simulink model "chap05"  (R2021a)
settings: Solver=FixedStepDiscrete  StartTime=0.0  StopTime=inf  FixedStep=0.001  RelTol=1e-3
undefined symbols (not defined in the file): DiscIntNeverNeededParam, Header, Pose, X, Y, Z
libraries: robotlib x31
(part 6 of 9)

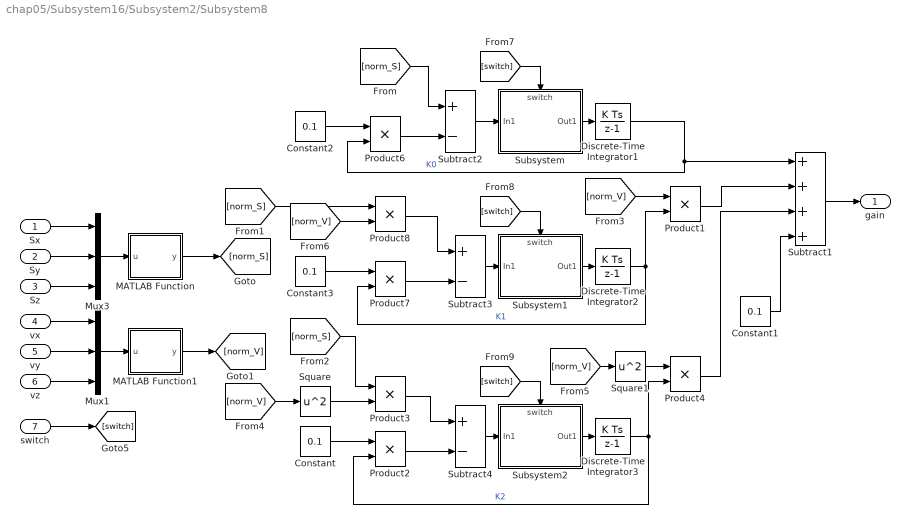
== system chap05/Subsystem16/Subsystem2/Subsystem8 ==
  Sx : Inport
  Sy : Inport  Port=2
  Sz : Inport  Port=3
  vx : Inport  Port=4
  vy : Inport  Port=5
  vz : Inport  Port=6
  switch : Inport  Port=7
  Constant{,1..3} (4 alike) : Constant  Value=0.1
  Discrete-Time Integrator1 : DiscreteIntegrator  gainval=1  InitialCondition=0.05  SampleTime=-1  ICPrevOutput=DiscIntNeverNeededParam  ICPrevScaledInput=DiscIntNeverNeededParam
  Discrete-Time Integrator2 : DiscreteIntegrator  gainval=1  InitialCondition=0.025  SampleTime=-1  ICPrevOutput=DiscIntNeverNeededParam  ICPrevScaledInput=DiscIntNeverNeededParam
  Discrete-Time Integrator3 : DiscreteIntegrator  gainval=1  InitialCondition=0.01  SampleTime=-1  ICPrevOutput=DiscIntNeverNeededParam  ICPrevScaledInput=DiscIntNeverNeededParam
  MATLAB Function : MATLAB Function  TreatAsAtomicUnit=on
  MATLAB Function1 : MATLAB Function  TreatAsAtomicUnit=on
  Mux1 : Mux  Inputs=3
  Mux3 : Mux  Inputs=3
  Product{1..4,6..8} (7 alike) : Product
  Square : Math  Operator=square  SaturateOnIntegerOverflow=on
  Square1 : Math  Operator=square  SaturateOnIntegerOverflow=on
  Subsystem : Subsystem
      settings: PortSchema="{\"entries\":[{\"content\":{\"sides\":[{\"content\":{\"connectorIds\":[\"In1\"]},\"type\":\"ConnectorPlacement.EquallySpacedRectSide\",\"uuid\":\"50b1559e-7173-4ba8-93e6-314f6d9df527\"},{\"content\":{\"connectorIds\":[\"Out1\"],\"side\":\"RIGHT\"},\"type\":\"ConnectorPlacement.EquallySpacedRectSide\",\"uuid\":\"be527bac-0bcc-4faf-a185-0382edae0189\"},{\"content\":{\"connectorIds\":[\"In2\"],\"side\":\"TOP\"},\"type\":\"ConnectorPlacement.EquallySpacedRectSide\",\"uuid\":\"4c8ef68d-7cf5-4d15-9758-89dbc1169805\"}]},\"type\":\"ConnectorPlacement.EquallySpacedConnector\",\"uuid\":\"3c2ee67b-c3c9-431a-8107-6d5cd22b236e\"}],\"packageUris\":[\"http://schema.mathworks.com/mf0/Connector/R2020b\"],\"version\":\"1.0\"}"
  Subsystem1 : Subsystem
      settings: PortSchema="{\"entries\":[{\"content\":{\"sides\":[{\"content\":{\"connectorIds\":[\"In1\"]},\"type\":\"ConnectorPlacement.EquallySpacedRectSide\",\"uuid\":\"50b1559e-7173-4ba8-93e6-314f6d9df527\"},{\"content\":{\"connectorIds\":[\"Out1\"],\"side\":\"RIGHT\"},\"type\":\"ConnectorPlacement.EquallySpacedRectSide\",\"uuid\":\"be527bac-0bcc-4faf-a185-0382edae0189\"},{\"content\":{\"connectorIds\":[\"In2\"],\"side\":\"TOP\"},\"type\":\"ConnectorPlacement.EquallySpacedRectSide\",\"uuid\":\"4c8ef68d-7cf5-4d15-9758-89dbc1169805\"}]},\"type\":\"ConnectorPlacement.EquallySpacedConnector\",\"uuid\":\"3c2ee67b-c3c9-431a-8107-6d5cd22b236e\"}],\"packageUris\":[\"http://schema.mathworks.com/mf0/Connector/R2020b\"],\"version\":\"1.0\"}"
  Subsystem2 : Subsystem
      settings: PortSchema="{\"entries\":[{\"content\":{\"sides\":[{\"content\":{\"connectorIds\":[\"In1\"]},\"type\":\"ConnectorPlacement.EquallySpacedRectSide\",\"uuid\":\"50b1559e-7173-4ba8-93e6-314f6d9df527\"},{\"content\":{\"connectorIds\":[\"Out1\"],\"side\":\"RIGHT\"},\"type\":\"ConnectorPlacement.EquallySpacedRectSide\",\"uuid\":\"be527bac-0bcc-4faf-a185-0382edae0189\"},{\"content\":{\"connectorIds\":[\"In2\"],\"side\":\"TOP\"},\"type\":\"ConnectorPlacement.EquallySpacedRectSide\",\"uuid\":\"4c8ef68d-7cf5-4d15-9758-89dbc1169805\"}]},\"type\":\"ConnectorPlacement.EquallySpacedConnector\",\"uuid\":\"3c2ee67b-c3c9-431a-8107-6d5cd22b236e\"}],\"packageUris\":[\"http://schema.mathworks.com/mf0/Connector/R2020b\"],\"version\":\"1.0\"}"
  Subtract1 : Sum  Inputs=++++
  Subtract2 : Sum  Inputs=+-
  Subtract3 : Sum  Inputs=+-
  Subtract4 : Sum  Inputs=+-
  " gain" : Outport
  wires:
  [switch] -> Subsystem2/2(switch)
  [switch] -> Subsystem1/2(switch)
  [switch] -> Subsystem/2(switch)
  switch/1 -> [switch]
  Subsystem1/1(Out1) -> Discrete-Time Integrator2/1
  Subsystem2/1(Out1) -> Discrete-Time Integrator3/1
  Subsystem/1(Out1) -> Discrete-Time Integrator1/1
  [norm_V] -> Product8/2
  Square1/1 -> Product4/1
  [norm_V] -> Square1/1
  [norm_V] -> Product1/1
  [norm_V] -> Square/1
  [norm_S] -> Product3/1
  [norm_S] -> Product8/1
  [norm_S] -> Subtract2/1
  MATLAB Function/1(y) -> [norm_S]
  vy/1 -> Mux1/2
  vz/1 -> Mux1/3
  vx/1 -> Mux1/1
  Sz/1 -> Mux3/3
  Sy/1 -> Mux3/2
  Sx/1 -> Mux3/1
  Constant3/1 -> Product7/1
  Constant2/1 -> Product6/1
  Constant1/1 -> Subtract1/4
  Product4/1 -> Subtract1/3
  MATLAB Function1/1(y) -> [norm_V]
  Constant/1 -> Product2/1
  Mux1/1 -> MATLAB Function1/1(u)
  Square/1 -> Product3/2
  Mux3/1 -> MATLAB Function/1(u)
  Discrete-Time Integrator3/1 -> Product2/2, Product4/2  "K2"
  Product2/1 -> Subtract4/2
  Product3/1 -> Subtract4/1
  Subtract4/1 -> Subsystem2/1(In1)
  Subtract3/1 -> Subsystem1/1(In1)
  Product8/1 -> Subtract3/1
  Product7/1 -> Subtract3/2
  Discrete-Time Integrator2/1 -> Product1/2, Product7/2  "K1"
  Product6/1 -> Subtract2/2
  Discrete-Time Integrator1/1 -> Subtract1/1, Product6/2  "K0"
  Subtract2/1 -> Subsystem/1(In1)
  Product1/1 -> Subtract1/2
  Subtract1/1 -> " gain"/1

== system chap05/Subsystem16/Subsystem2/Subsystem9 ==
  vy2 : Inport
  uty : Inport  Port=2
  gain : Inport  Port=3
  switch : Inport  Port=4
  Add1 : Sum  Inputs=--+
  Constant1 : Constant  Value=0.08
  Constant2 : Constant  Value=10
  Product : Product
  Product1 : Product
  Product2 : Product
  Subsystem : Subsystem
  Subtract : Sum  Inputs=+-
  Switch1 : Switch  Criteria=u2 > Threshold  Threshold=1
  Tanh : Trigonometry  Operator=tanh
  uy : Outport
  Sz : Outport  Port=2
  wires:
  Switch1/1 -> uy/1
  [switch] -> Switch1/2
  [A] -> Switch1/3
  switch/1 -> Subsystem/1(switch), [switch]
  Subtract/1 -> Product2/1, Product1/2, Sz/1
  Product1/1 -> Add1/1
  Constant2/1 -> Product2/2
  [A] -> Add1/3
  gain/1 -> Product/2
  Tanh/1 -> Product/1
  Product2/1 -> Tanh/1
  vy2/1 -> Subtract/1
  Product/1 -> Add1/2
  uty/1 -> Subsystem/2(zt3), [A]
  Add1/1 -> Switch1/1
  Subsystem/1(Out1) -> Subtract/2
  Constant1/1 -> Product1/1

== system chap05/Subsystem16/Subsystem3/Subsystem1 ==
  xy4 : Inport
  xy2 : Inport  Port=2
  xy3 : Inport  Port=3
  xy5 : Inport  Port=4
  vy4 : Inport  Port=5
  vy2 : Inport  Port=6
  vy3 : Inport  Port=7
  vy5 : Inport  Port=8
  Add : Sum
  Add{1,4,6,8} (4 alike) : Sum  Inputs=-+
  Add2 : Sum  Inputs=+-
  Add5 : Sum  Inputs=+++
  Add7 : Sum  Inputs=+-
  Add9 : Sum  Inputs=+++
  Constant : Constant  Value=0.75
  Constant1 : Constant  Value=0.85
  Constant2 : Constant  Value=0.8
  Constant3 : Constant  Value=0.8
  Constant4 : Constant  Value=0.5
  Constant5 : Constant  Value=1.2
  Constant6 : Constant  Value=0.5
  Constant7 : Constant  Value=1.2
  Gain : Gain  Gain=-1
  Product{1,3..9} (8 alike) : Product
  utx : Outport
  wires:
  Add9/1 -> Product1/2
  Product4/1 -> Add5/2
  Product5/1 -> Add5/3
  Constant3/1 -> Product4/1
  Add4/1 -> Product4/2
  xy4/1 -> Add1/2, Add4/2, Add2/1
  Constant4/1 -> Product5/2
  Product6/1 -> Add/1
  Constant/1 -> Product6/1
  Constant1/1 -> Product1/1
  Product1/1 -> Add/2
  Add2/1 -> Product5/1
  Add5/1 -> Product6/2
  xy3/1 -> Add4/1
  xy2/1 -> Add2/2
  xy5/1 -> Add1/1
  Constant5/1 -> Product3/1
  Add1/1 -> Product3/2
  Product3/1 -> Add5/1
  Product7/1 -> Add9/1
  Add6/1 -> Product7/2
  Constant7/1 -> Product7/1
  vy5/1 -> Add6/1
  vy2/1 -> Add7/2
  vy3/1 -> Add8/1
  Add7/1 -> Product9/1
  Constant6/1 -> Product9/2
  vy4/1 -> Add7/1, Add8/2, Add6/2
  Add8/1 -> Product8/2
  Constant2/1 -> Product8/1
  Product9/1 -> Add9/3
  Product8/1 -> Add9/2
  Gain/1 -> utx/1
  Add/1 -> Gain/1

== system chap05/Subsystem16/Subsystem3/Subsystem10 ==
  utx : Inport
  uty : Inport  Port=2
  utz : Inport  Port=3
  Add : Sum
  Constant3 : Constant
  Constant4 : Constant  Value=0
  Data Store Memory : DataStoreMemory  DataStoreName=utkz4  ReadBeforeWriteMsg=warning  WriteAfterWriteMsg=warning  WriteAfterReadMsg=warning  ShowAdditionalParam=off
  Data Store Memory1 : DataStoreMemory  DataStoreName=utky4  ReadBeforeWriteMsg=warning  WriteAfterWriteMsg=warning  WriteAfterReadMsg=warning  ShowAdditionalParam=off
  Data Store Memory2 : DataStoreMemory  DataStoreName=utkx4  ReadBeforeWriteMsg=warning  WriteAfterWriteMsg=warning  WriteAfterReadMsg=warning  ShowAdditionalParam=off
  Data Store Memory3 : DataStoreMemory  DataStoreName=uc4  ReadBeforeWriteMsg=warning  WriteAfterWriteMsg=warning  WriteAfterReadMsg=warning  ShowAdditionalParam=off
  Data Store Read : DataStoreRead  DataStoreName=uc4  IndexOptions=Index vector (dialog)  Indices=1  OutputSizes=1
  Data Store Read1 : DataStoreRead  DataStoreName=utkz4  IndexOptions=Index vector (dialog)  Indices=1  OutputSizes=1
  Data Store Read2 : DataStoreRead  DataStoreName=utky4  IndexOptions=Index vector (dialog)  Indices=1  OutputSizes=1
  Data Store Read3 : DataStoreRead  DataStoreName=utkx4  IndexOptions=Index vector (dialog)  Indices=1  OutputSizes=1
  Data Store Write : DataStoreWrite  DataStoreName=uc4  IndexOptions=Index vector (dialog)  Indices=1  OutputSizes=1
  Data Store Write3 : DataStoreWrite  DataStoreName=utkx4  IndexOptions=Index vector (dialog)  Indices=1  OutputSizes=1
  Data Store Write4 : DataStoreWrite  DataStoreName=utky4  IndexOptions=Index vector (dialog)  Indices=1  OutputSizes=1
  Data Store Write5 : DataStoreWrite  DataStoreName=utkz4  IndexOptions=Index vector (dialog)  Indices=1  OutputSizes=1
  Demux : Demux  Outputs=3
  Display : Display
  MATLAB Function : MATLAB Function  TreatAsAtomicUnit=on
  Mux1 : Mux  Inputs=3
  Mux2 : Mux  Inputs=3
  Switch : Switch  Threshold=0.1
  Switch2 : Switch  Threshold=0.1
  ux : Outport
  uy : Outport  Port=2
  uz : Outport  Port=3
  wires:
  Mux2/1 -> [utk], MATLAB Function/2(utk)
  Mux1/1 -> [ut], MATLAB Function/1(u)
  Switch/1 -> Demux/1
  Data Store Read3/1 -> Mux2/1
  Data Store Read1/1 -> Mux2/3
  Data Store Read2/1 -> Mux2/2
  Demux/3 -> Data Store Write5/1, uz/1
  Demux/1 -> Data Store Write3/1, ux/1
  Add/1 -> Data Store Write/1, Display/1
  Data Store Read/1 -> Add/2
  Switch2/1 -> Add/1  "e1"
  Constant3/1 -> Switch2/1
  Constant4/1 -> Switch2/3
  MATLAB Function/1(nrom) -> Switch2/2, Switch/2
  utx/1 -> Mux1/1
  uty/1 -> Mux1/2
  utz/1 -> Mux1/3
  Demux/2 -> Data Store Write4/1, uy/1
  [ut] -> Switch/1
  [utk] -> Switch/3

== system chap05/Subsystem16/Subsystem3/Subsystem11 ==
  vz4 : Inport
  utz : Inport  Port=2
  gain : Inport  Port=3
  switch : Inport  Port=4
  Add1 : Sum  Inputs=--+
  Constant1 : Constant  Value=0.08
  Constant2 : Constant  Value=10
  Product : Product
  Product1 : Product
  Product2 : Product
  Subsystem : Subsystem
  Subtract : Sum  Inputs=+-
  Switch1 : Switch  Criteria=u2 > Threshold  Threshold=1
  Tanh : Trigonometry  Operator=tanh
  uz : Outport
  Sz : Outport  Port=2
  wires:
  Add1/1 -> Switch1/1
  utz/1 -> [A], Subsystem/2(zt3)
  Product/1 -> Add1/2
  vz4/1 -> Subtract/1
  Product2/1 -> Tanh/1
  Tanh/1 -> Product/1
  gain/1 -> Product/2
  [A] -> Add1/3
  Constant2/1 -> Product2/2
  Product1/1 -> Add1/1
  Constant1/1 -> Product1/1
  Subtract/1 -> Sz/1, Product1/2, Product2/1
  Subsystem/1(Out1) -> Subtract/2
  switch/1 -> [switch], Subsystem/1(switch)
  [A] -> Switch1/3
  [switch] -> Switch1/2
  Switch1/1 -> uz/1

== system chap05/Subsystem16/Subsystem3/Subsystem2 ==
  xz4 : Inport
  xx2 : Inport  Port=2
  xz3 : Inport  Port=3
  xz5 : Inport  Port=4
  vz4 : Inport  Port=5
  vz2 : Inport  Port=6
  vz3 : Inport  Port=7
  vz5 : Inport  Port=8
  Add : Sum
  Add{1,4,6,8} (4 alike) : Sum  Inputs=-+
  Add2 : Sum  Inputs=+-
  Add5 : Sum  Inputs=+++
  Add7 : Sum  Inputs=+-
  Add9 : Sum  Inputs=+++
  Constant : Constant  Value=0.75
  Constant1 : Constant  Value=0.85
  Constant2 : Constant  Value=0.8
  Constant3 : Constant  Value=0.8
  Constant4 : Constant  Value=0.5
  Constant5 : Constant  Value=1.2
  Constant6 : Constant  Value=0.5
  Constant7 : Constant  Value=1.2
  Gain : Gain  Gain=-1
  Product{1,3..9} (8 alike) : Product
  utx : Outport
  wires:
  Product8/1 -> Add9/2
  Product9/1 -> Add9/3
  Constant2/1 -> Product8/1
  Add8/1 -> Product8/2
  vz4/1 -> Add6/2, Add8/2, Add7/1
  Constant6/1 -> Product9/2
  Add7/1 -> Product9/1
  vz3/1 -> Add8/1
  vz2/1 -> Add7/2
  vz5/1 -> Add6/1
  Constant7/1 -> Product7/1
  Add6/1 -> Product7/2
  Product7/1 -> Add9/1
  Product3/1 -> Add5/1
  Add1/1 -> Product3/2
  Constant5/1 -> Product3/1
  xz5/1 -> Add1/1
  xx2/1 -> Add2/2
  xz3/1 -> Add4/1
  Add5/1 -> Product6/2
  Add2/1 -> Product5/1
  Product1/1 -> Add/2
  Constant1/1 -> Product1/1
  Constant/1 -> Product6/1
  Product6/1 -> Add/1
  Constant4/1 -> Product5/2
  xz4/1 -> Add2/1, Add4/2, Add1/2
  Add4/1 -> Product4/2
  Constant3/1 -> Product4/1
  Product5/1 -> Add5/3
  Product4/1 -> Add5/2
  Add9/1 -> Product1/2
  Gain/1 -> utx/1
  Add/1 -> Gain/1

== system chap05/Subsystem16/Subsystem3/Subsystem3 ==
  utx : Inport
  vx : Inport  Port=2
  vy : Inport  Port=3
  vz : Inport  Port=4
  uty : Inport  Port=5
  ux : Inport  Port=6
  uy : Inport  Port=7
  uz : Inport  Port=8
  utz : Inport  Port=9
  switch : Inport  Port=10
  Add3 : Sum  Inputs=-+
  Add4 : Sum  Inputs=-+
  Add5 : Sum  Inputs=-+
  Demux : Demux  Outputs=3
  Demux1 : Demux  Outputs=3
  Discrete-Time Integrator1 : DiscreteIntegrator  SampleTime=-1  ICPrevOutput=DiscIntNeverNeededParam  ICPrevScaledInput=DiscIntNeverNeededParam
  Discrete-Time Integrator2 : DiscreteIntegrator  SampleTime=-1  ICPrevOutput=DiscIntNeverNeededParam  ICPrevScaledInput=DiscIntNeverNeededParam
  Discrete-Time Integrator8 : DiscreteIntegrator  SampleTime=-1  ICPrevOutput=DiscIntNeverNeededParam  ICPrevScaledInput=DiscIntNeverNeededParam
  MATLAB Function : MATLAB Function  TreatAsAtomicUnit=on
  MATLAB Function1 : MATLAB Function  TreatAsAtomicUnit=on
  MATLAB Function2 : MATLAB Function  TreatAsAtomicUnit=on
  Mux : Mux  Inputs=3
  Mux1 : Mux  Inputs=3
  Subsystem : Subsystem
  Subsystem1 : Subsystem
  Subsystem2 : Subsystem
      settings: PortSchema="{\"entries\":[{\"content\":{\"sides\":[{\"content\":{\"connectorIds\":[\"In1\"]},\"type\":\"ConnectorPlacement.EquallySpacedRectSide\",\"uuid\":\"fc08b57d-5108-4bb3-894e-d1527c9ee9b9\"},{\"content\":{\"connectorIds\":[\"Out1\",\"Out2\",\"Out3\",\"Out4\"],\"side\":\"RIGHT\"},\"type\":\"ConnectorPlacement.EquallySpacedRectSide\",\"uuid\":\"5f28f464-9d6d-4ee7-848e-113b4b51ead6\"},{\"content\":{\"connectorIds\":[],\"side\":\"TOP\"},\"type\":\"ConnectorPlacement.EquallySpacedRectSide\",\"uuid\":\"5cca314e-822b-43eb-ac4d-78622e8ed582\"},{\"content\":{\"connectorIds\":[\"In2\"],\"side\":\"BOTTOM\"},\"type\":\"ConnectorPlacement.EquallySpacedRectSide\",\"uuid\":\"aa07b2d0-4f6e-4d8e-96de-14c35ee3da88\"}]},\"type\":\"ConnectorPlacement.EquallySpacedConnector\",\"uuid\":\"246d6f2c-2f9e-403c-b810-eff9b0fc0735\"}],\"packageUris\":[\"http://schema.mathworks.com/mf0/Connector/R2020b\"],\"version\":\"1.0\"}"
  Subsystem3 : Subsystem
  Subtract1 : Sum  Inputs=++++
  Subtract2 : Sum  Inputs=+-
  Subtract3 : Sum  Inputs=+-
  Subtract4 : Sum  Inputs=+-
  Switch1 : Switch  Criteria=u2 > Threshold  Threshold=1
  Switch2 : Switch  Criteria=u2 > Threshold  Threshold=1
  Switch3 : Switch  Criteria=u2 > Threshold  Threshold=1
  udtx : Outport
  udty : Outport  Port=2
  udtz : Outport  Port=3
  wires:
  Subsystem3/1(Out1) -> Subtract1/2
  Subsystem2/2(k2) -> Subsystem3/2(k2)
  Subsystem1/1(Out1) -> Subtract1/1
  Subsystem2/1(k1) -> Subsystem1/2(k1)
  Subtract4/1 -> MATLAB Function2/1(u)
  Subtract3/1 -> MATLAB Function1/1(u)
  Subtract2/1 -> MATLAB Function/1(u)
  Demux/3 -> Discrete-Time Integrator8/1
  Demux/1 -> Discrete-Time Integrator2/1
  Demux/2 -> Discrete-Time Integrator1/1
  Discrete-Time Integrator2/1 -> Subtract2/1
  Discrete-Time Integrator1/1 -> Subtract3/1
  Discrete-Time Integrator8/1 -> Subtract4/1
  Mux1/1 -> Subtract1/4
  ux/1 -> Mux1/1
  uy/1 -> Mux1/2
  uz/1 -> Mux1/3
  vx/1 -> Subtract2/2
  Subsystem2/4(k4) -> Subsystem/3(k4)
  Subsystem/1(z2) -> Subtract1/3, Demux1/1  "od4"
  Subsystem2/3(k3) -> Subsystem/2(k3)
  Subtract1/1 -> Demux/1
  Mux/1 -> Subsystem1/1(e1), Subsystem3/1(e1), Subsystem2/1(e1), Subsystem/1(e1)
  utx/1 -> Switch1/3, Add3/2
  uty/1 -> Switch2/3, Add5/2
  utz/1 -> Switch3/3, Add4/2
  vy/1 -> Subtract3/2
  vz/1 -> Subtract4/2
  MATLAB Function/1(y) -> Mux/1
  MATLAB Function1/1(y) -> Mux/2
  MATLAB Function2/1(y) -> Mux/3
  switch/1 -> [switch], Switch3/2, Switch2/2, Switch1/2
  [switch] -> Subsystem2/2(switch)
  Add3/1 -> Switch1/1
  Add5/1 -> Switch2/1
  Add4/1 -> Switch3/1
  Switch1/1 -> udtx/1
  Switch2/1 -> udty/1
  Switch3/1 -> udtz/1
  Demux1/1 -> Add3/1
  Demux1/2 -> Add5/1
  Demux1/3 -> Add4/1

== system chap05/Subsystem16/Subsystem3/Subsystem4 ==
  vx4 : Inport
  utx : Inport  Port=2
  gain : Inport  Port=3
  switch : Inport  Port=4
  Add1 : Sum  Inputs=--+
  Constant1 : Constant  Value=0.08
  Constant2 : Constant  Value=10
  Product : Product
  Product1 : Product
  Product2 : Product
  Subsystem : Subsystem
  Subtract : Sum  Inputs=+-
  Switch1 : Switch  Criteria=u2 > Threshold  Threshold=1
  Tanh : Trigonometry  Operator=tanh
  ux : Outport
  Sx : Outport  Port=2
  wires:
  Add1/1 -> Switch1/1
  utx/1 -> [A], Subsystem/2(zt3)
  Product/1 -> Add1/2
  vx4/1 -> Subtract/1
  Product2/1 -> Tanh/1
  Tanh/1 -> Product/1
  gain/1 -> Product/2
  [A] -> Add1/3
  Constant2/1 -> Product2/2
  Product1/1 -> Add1/1
  Constant1/1 -> Product1/1
  Subtract/1 -> Sx/1, Product1/2, Product2/1
  switch/1 -> [switch], Subsystem/1(switch)
  [A] -> Switch1/3
  [switch] -> Switch1/2
  Switch1/1 -> ux/1
  Subsystem/1(Out1) -> Subtract/2

== system chap05/Subsystem16/Subsystem3/Subsystem6 ==
  xx4 : Inport
  xx2 : Inport  Port=2
  xx3 : Inport  Port=3
  xx5 : Inport  Port=4
  vx4 : Inport  Port=5
  vx2 : Inport  Port=6
  vx3 : Inport  Port=7
  vx5 : Inport  Port=8
  Add : Sum
  Add{1,4,6,8} (4 alike) : Sum  Inputs=-+
  Add2 : Sum  Inputs=+-
  Add5 : Sum  Inputs=+++
  Add7 : Sum  Inputs=+-
  Add9 : Sum  Inputs=+++
  Constant : Constant  Value=0.75
  Constant1 : Constant  Value=0.85
  Constant2 : Constant  Value=0.8
  Constant3 : Constant  Value=0.8
  Constant4 : Constant  Value=0.5
  Constant5 : Constant  Value=1.2
  Constant6 : Constant  Value=0.5
  Constant7 : Constant  Value=1.2
  Gain : Gain  Gain=-1
  Product{1,3..9} (8 alike) : Product
  utx : Outport
  wires:
  Product8/1 -> Add9/2
  Product9/1 -> Add9/3
  Constant2/1 -> Product8/1
  Add8/1 -> Product8/2
  vx4/1 -> Add6/2, Add8/2, Add7/1
  Constant6/1 -> Product9/2
  Add7/1 -> Product9/1
  vx3/1 -> Add8/1
  vx2/1 -> Add7/2
  vx5/1 -> Add6/1
  Constant7/1 -> Product7/1
  Add6/1 -> Product7/2
  Product7/1 -> Add9/1
  Product3/1 -> Add5/1
  Add1/1 -> Product3/2
  Constant5/1 -> Product3/1
  xx5/1 -> Add1/1
  xx2/1 -> Add2/2
  xx3/1 -> Add4/1
  Add5/1 -> Product6/2
  Add2/1 -> Product5/1
  Product1/1 -> Add/2
  Constant1/1 -> Product1/1
  Constant/1 -> Product6/1
  Product6/1 -> Add/1
  Constant4/1 -> Product5/2
  xx4/1 -> Add2/1, Add4/2, Add1/2
  Add4/1 -> Product4/2
  Constant3/1 -> Product4/1
  Product5/1 -> Add5/3
  Product4/1 -> Add5/2
  Add9/1 -> Product1/2
  Gain/1 -> utx/1
  Add/1 -> Gain/1

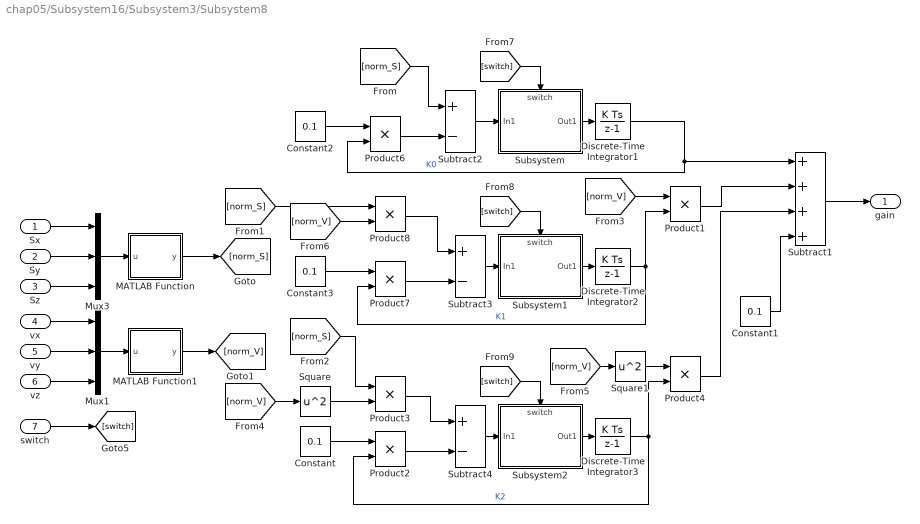
== system chap05/Subsystem16/Subsystem3/Subsystem8 ==
  Sx : Inport
  Sy : Inport  Port=2
  Sz : Inport  Port=3
  vx : Inport  Port=4
  vy : Inport  Port=5
  vz : Inport  Port=6
  switch : Inport  Port=7
  Constant{,1..3} (4 alike) : Constant  Value=0.1
  Discrete-Time Integrator1 : DiscreteIntegrator  gainval=1  InitialCondition=0.05  SampleTime=-1  ICPrevOutput=DiscIntNeverNeededParam  ICPrevScaledInput=DiscIntNeverNeededParam
  Discrete-Time Integrator2 : DiscreteIntegrator  gainval=1  InitialCondition=0.025  SampleTime=-1  ICPrevOutput=DiscIntNeverNeededParam  ICPrevScaledInput=DiscIntNeverNeededParam
  Discrete-Time Integrator3 : DiscreteIntegrator  gainval=1  InitialCondition=0.01  SampleTime=-1  ICPrevOutput=DiscIntNeverNeededParam  ICPrevScaledInput=DiscIntNeverNeededParam
  MATLAB Function : MATLAB Function  TreatAsAtomicUnit=on
  MATLAB Function1 : MATLAB Function  TreatAsAtomicUnit=on
  Mux1 : Mux  Inputs=3
  Mux3 : Mux  Inputs=3
  Product{1..4,6..8} (7 alike) : Product
  Square : Math  Operator=square  SaturateOnIntegerOverflow=on
  Square1 : Math  Operator=square  SaturateOnIntegerOverflow=on
  Subsystem : Subsystem
      settings: PortSchema="{\"entries\":[{\"content\":{\"sides\":[{\"content\":{\"connectorIds\":[\"In1\"]},\"type\":\"ConnectorPlacement.EquallySpacedRectSide\",\"uuid\":\"50b1559e-7173-4ba8-93e6-314f6d9df527\"},{\"content\":{\"connectorIds\":[\"Out1\"],\"side\":\"RIGHT\"},\"type\":\"ConnectorPlacement.EquallySpacedRectSide\",\"uuid\":\"be527bac-0bcc-4faf-a185-0382edae0189\"},{\"content\":{\"connectorIds\":[\"In2\"],\"side\":\"TOP\"},\"type\":\"ConnectorPlacement.EquallySpacedRectSide\",\"uuid\":\"4c8ef68d-7cf5-4d15-9758-89dbc1169805\"}]},\"type\":\"ConnectorPlacement.EquallySpacedConnector\",\"uuid\":\"3c2ee67b-c3c9-431a-8107-6d5cd22b236e\"}],\"packageUris\":[\"http://schema.mathworks.com/mf0/Connector/R2020b\"],\"version\":\"1.0\"}"
  Subsystem1 : Subsystem
      settings: PortSchema="{\"entries\":[{\"content\":{\"sides\":[{\"content\":{\"connectorIds\":[\"In1\"]},\"type\":\"ConnectorPlacement.EquallySpacedRectSide\",\"uuid\":\"50b1559e-7173-4ba8-93e6-314f6d9df527\"},{\"content\":{\"connectorIds\":[\"Out1\"],\"side\":\"RIGHT\"},\"type\":\"ConnectorPlacement.EquallySpacedRectSide\",\"uuid\":\"be527bac-0bcc-4faf-a185-0382edae0189\"},{\"content\":{\"connectorIds\":[\"In2\"],\"side\":\"TOP\"},\"type\":\"ConnectorPlacement.EquallySpacedRectSide\",\"uuid\":\"4c8ef68d-7cf5-4d15-9758-89dbc1169805\"}]},\"type\":\"ConnectorPlacement.EquallySpacedConnector\",\"uuid\":\"3c2ee67b-c3c9-431a-8107-6d5cd22b236e\"}],\"packageUris\":[\"http://schema.mathworks.com/mf0/Connector/R2020b\"],\"version\":\"1.0\"}"
  Subsystem2 : Subsystem
      settings: PortSchema="{\"entries\":[{\"content\":{\"sides\":[{\"content\":{\"connectorIds\":[\"In1\"]},\"type\":\"ConnectorPlacement.EquallySpacedRectSide\",\"uuid\":\"50b1559e-7173-4ba8-93e6-314f6d9df527\"},{\"content\":{\"connectorIds\":[\"Out1\"],\"side\":\"RIGHT\"},\"type\":\"ConnectorPlacement.EquallySpacedRectSide\",\"uuid\":\"be527bac-0bcc-4faf-a185-0382edae0189\"},{\"content\":{\"connectorIds\":[\"In2\"],\"side\":\"TOP\"},\"type\":\"ConnectorPlacement.EquallySpacedRectSide\",\"uuid\":\"4c8ef68d-7cf5-4d15-9758-89dbc1169805\"}]},\"type\":\"ConnectorPlacement.EquallySpacedConnector\",\"uuid\":\"3c2ee67b-c3c9-431a-8107-6d5cd22b236e\"}],\"packageUris\":[\"http://schema.mathworks.com/mf0/Connector/R2020b\"],\"version\":\"1.0\"}"
  Subtract1 : Sum  Inputs=++++
  Subtract2 : Sum  Inputs=+-
  Subtract3 : Sum  Inputs=+-
  Subtract4 : Sum  Inputs=+-
  " gain" : Outport
  wires:
  [switch] -> Subsystem2/2(switch)
  [switch] -> Subsystem1/2(switch)
  [switch] -> Subsystem/2(switch)
  switch/1 -> [switch]
  Subsystem1/1(Out1) -> Discrete-Time Integrator2/1
  Subsystem2/1(Out1) -> Discrete-Time Integrator3/1
  Subsystem/1(Out1) -> Discrete-Time Integrator1/1
  [norm_V] -> Product8/2
  Square1/1 -> Product4/1
  [norm_V] -> Square1/1
  [norm_V] -> Product1/1
  [norm_V] -> Square/1
  [norm_S] -> Product3/1
  [norm_S] -> Product8/1
  [norm_S] -> Subtract2/1
  MATLAB Function/1(y) -> [norm_S]
  vy/1 -> Mux1/2
  vz/1 -> Mux1/3
  vx/1 -> Mux1/1
  Sz/1 -> Mux3/3
  Sy/1 -> Mux3/2
  Sx/1 -> Mux3/1
  Constant3/1 -> Product7/1
  Constant2/1 -> Product6/1
  Constant1/1 -> Subtract1/4
  Product4/1 -> Subtract1/3
  MATLAB Function1/1(y) -> [norm_V]
  Constant/1 -> Product2/1
  Mux1/1 -> MATLAB Function1/1(u)
  Square/1 -> Product3/2
  Mux3/1 -> MATLAB Function/1(u)
  Discrete-Time Integrator3/1 -> Product2/2, Product4/2  "K2"
  Product2/1 -> Subtract4/2
  Product3/1 -> Subtract4/1
  Subtract4/1 -> Subsystem2/1(In1)
  Subtract3/1 -> Subsystem1/1(In1)
  Product8/1 -> Subtract3/1
  Product7/1 -> Subtract3/2
  Discrete-Time Integrator2/1 -> Product1/2, Product7/2  "K1"
  Product6/1 -> Subtract2/2
  Discrete-Time Integrator1/1 -> Subtract1/1, Product6/2  "K0"
  Subtract2/1 -> Subsystem/1(In1)
  Product1/1 -> Subtract1/2
  Subtract1/1 -> " gain"/1

== system chap05/Subsystem16/Subsystem3/Subsystem9 ==
  vy4 : Inport
  uty : Inport  Port=2
  gain : Inport  Port=3
  switch : Inport  Port=4
  Add1 : Sum  Inputs=--+
  Constant1 : Constant  Value=0.08
  Constant2 : Constant  Value=10
  Product : Product
  Product1 : Product
  Product2 : Product
  Subsystem : Subsystem
  Subtract : Sum  Inputs=+-
  Switch1 : Switch  Criteria=u2 > Threshold  Threshold=1
  Tanh : Trigonometry  Operator=tanh
  uy : Outport
  Sz : Outport  Port=2
  wires:
  Switch1/1 -> uy/1
  [switch] -> Switch1/2
  [A] -> Switch1/3
  switch/1 -> Subsystem/1(switch), [switch]
  Subtract/1 -> Product2/1, Product1/2, Sz/1
  Constant1/1 -> Product1/1
  Product1/1 -> Add1/1
  Constant2/1 -> Product2/2
  [A] -> Add1/3
  gain/1 -> Product/2
  Tanh/1 -> Product/1
  Product2/1 -> Tanh/1
  vy4/1 -> Subtract/1
  Product/1 -> Add1/2
  uty/1 -> Subsystem/2(zt3), [A]
  Add1/1 -> Switch1/1
  Subsystem/1(Out1) -> Subtract/2

== system chap05/Subsystem16/Subsystem5/Subsystem1 ==
  xy3 : Inport
  xy1 : Inport  Port=2
  xy4 : Inport  Port=3
  xy5 : Inport  Port=4
  vy3 : Inport  Port=5
  vy1 : Inport  Port=6
  vy4 : Inport  Port=7
  vy5 : Inport  Port=8
  Add : Sum
  Add{1,4,6,8} (4 alike) : Sum  Inputs=-+
  Add2 : Sum  Inputs=+-
  Add5 : Sum  Inputs=+++
  Add7 : Sum  Inputs=+-
  Add9 : Sum  Inputs=+++
  Constant : Constant  Value=0.75
  Constant1 : Constant  Value=0.85
  Constant2 : Constant  Value=0.8
  Constant3 : Constant  Value=0.8
  Constant4 : Constant  Value=0.5
  Constant5 : Constant  Value=1.5
  Constant6 : Constant  Value=0.5
  Constant7 : Constant  Value=1.5
  Gain : Gain  Gain=-1
  Product{1,3..9} (8 alike) : Product
  p3y : Outport
  wires:
  Add9/1 -> Product1/2
  Product4/1 -> Add5/2
  Product5/1 -> Add5/3
  Constant3/1 -> Product4/1
  Add4/1 -> Product4/2
  xy3/1 -> Add1/2, Add4/2, Add2/1
  Constant4/1 -> Product5/2
  Product6/1 -> Add/1
  Constant/1 -> Product6/1
  Constant1/1 -> Product1/1
  Product1/1 -> Add/2
  Add2/1 -> Product5/1
  Add5/1 -> Product6/2
  xy4/1 -> Add4/1
  xy1/1 -> Add2/2
  xy5/1 -> Add1/1
  Constant5/1 -> Product3/1
  Add1/1 -> Product3/2
  Product3/1 -> Add5/1
  Product7/1 -> Add9/1
  Add6/1 -> Product7/2
  Constant7/1 -> Product7/1
  vy5/1 -> Add6/1
  vy1/1 -> Add7/2
  vy4/1 -> Add8/1
  Add7/1 -> Product9/1
  Constant6/1 -> Product9/2
  vy3/1 -> Add7/1, Add8/2, Add6/2
  Add8/1 -> Product8/2
  ? -> Product8/1
  Product9/1 -> Add9/3
  Product8/1 -> Add9/2
  Gain/1 -> p3y/1
  Add/1 -> Gain/1

== system chap05/Subsystem16/Subsystem5/Subsystem10 ==
  utx : Inport
  uty : Inport  Port=2
  utz : Inport  Port=3
  Add : Sum
  Constant3 : Constant
  Constant4 : Constant  Value=0
  Data Store Memory : DataStoreMemory  DataStoreName=utkz3  ReadBeforeWriteMsg=warning  WriteAfterWriteMsg=warning  WriteAfterReadMsg=warning  ShowAdditionalParam=off
  Data Store Memory1 : DataStoreMemory  DataStoreName=utky3  ReadBeforeWriteMsg=warning  WriteAfterWriteMsg=warning  WriteAfterReadMsg=warning  ShowAdditionalParam=off
  Data Store Memory2 : DataStoreMemory  DataStoreName=utkx3  ReadBeforeWriteMsg=warning  WriteAfterWriteMsg=warning  WriteAfterReadMsg=warning  ShowAdditionalParam=off
  Data Store Memory3 : DataStoreMemory  DataStoreName=uc3  ReadBeforeWriteMsg=warning  WriteAfterWriteMsg=warning  WriteAfterReadMsg=warning  ShowAdditionalParam=off
  Data Store Read : DataStoreRead  DataStoreName=uc3  IndexOptions=Index vector (dialog)  Indices=1  OutputSizes=1
  Data Store Read4 : DataStoreRead  DataStoreName=utky3  IndexOptions=Index vector (dialog)  Indices=1  OutputSizes=1
  Data Store Read5 : DataStoreRead  DataStoreName=utkz3  IndexOptions=Index vector (dialog)  Indices=1  OutputSizes=1
  Data Store Read6 : DataStoreRead  DataStoreName=utkx3  IndexOptions=Index vector (dialog)  Indices=1  OutputSizes=1
  Data Store Write : DataStoreWrite  DataStoreName=uc3  IndexOptions=Index vector (dialog)  Indices=1  OutputSizes=1
  Data Store Write1 : DataStoreWrite  DataStoreName=utkx3  IndexOptions=Index vector (dialog)  Indices=1  OutputSizes=1
  Data Store Write2 : DataStoreWrite  DataStoreName=utky3  IndexOptions=Index vector (dialog)  Indices=1  OutputSizes=1
  Data Store Write3 : DataStoreWrite  DataStoreName=utkz3  IndexOptions=Index vector (dialog)  Indices=1  OutputSizes=1
  Demux : Demux  Outputs=3
  Display : Display
  MATLAB Function : MATLAB Function  TreatAsAtomicUnit=on
  Mux1 : Mux  Inputs=3
  Mux2 : Mux  Inputs=3
  Switch : Switch  Threshold=0.1
  Switch2 : Switch  Threshold=0.1
  ux : Outport
  uy : Outport  Port=2
  uz : Outport  Port=3
  wires:
  Mux2/1 -> [utk], MATLAB Function/2(utk)
  Mux1/1 -> [ut], MATLAB Function/1(u)
  Switch/1 -> Demux/1
  Data Store Read6/1 -> Mux2/1
  Data Store Read5/1 -> Mux2/3
  Data Store Read4/1 -> Mux2/2
  Demux/3 -> Data Store Write3/1, uz/1
  Demux/1 -> Data Store Write1/1, ux/1
  Add/1 -> Data Store Write/1, Display/1
  Data Store Read/1 -> Add/2
  Switch2/1 -> Add/1  "e1"
  Constant3/1 -> Switch2/1
  Constant4/1 -> Switch2/3
  MATLAB Function/1(nrom) -> Switch2/2, Switch/2
  utx/1 -> Mux1/1
  uty/1 -> Mux1/2
  utz/1 -> Mux1/3
  Demux/2 -> Data Store Write2/1, uy/1
  [ut] -> Switch/1
  [utk] -> Switch/3

== system chap05/Subsystem16/Subsystem5/Subsystem11 ==
  vz3 : Inport
  utz : Inport  Port=2
  gain : Inport  Port=3
  switch : Inport  Port=4
  Add1 : Sum  Inputs=--+
  Constant1 : Constant  Value=0.08
  Constant2 : Constant  Value=10
  Product : Product
  Product1 : Product
  Product2 : Product
  Subsystem : Subsystem
  Subtract : Sum  Inputs=+-
  Switch1 : Switch  Criteria=u2 > Threshold  Threshold=1
  Tanh : Trigonometry  Operator=tanh
  uz : Outport
  Sz : Outport  Port=2
  wires:
  Add1/1 -> Switch1/1
  utz/1 -> [A], Subsystem/2(zt3)
  Product/1 -> Add1/2
  vz3/1 -> Subtract/1
  Product2/1 -> Tanh/1
  Tanh/1 -> Product/1
  gain/1 -> Product/2
  [A] -> Add1/3
  Constant2/1 -> Product2/2
  Product1/1 -> Add1/1
  Constant1/1 -> Product1/1
  Subtract/1 -> Sz/1, Product1/2, Product2/1
  Subsystem/1(Out1) -> Subtract/2
  switch/1 -> [switch], Subsystem/1(switch)
  [A] -> Switch1/3
  [switch] -> Switch1/2
  Switch1/1 -> uz/1

== system chap05/Subsystem16/Subsystem5/Subsystem2 ==
  xz3 : Inport
  xz1 : Inport  Port=2
  xz4 : Inport  Port=3
  xz5 : Inport  Port=4
  vz3 : Inport  Port=5
  vz1 : Inport  Port=6
  vz4 : Inport  Port=7
  vz5 : Inport  Port=8
  Add : Sum
  Add{1,4,6,8} (4 alike) : Sum  Inputs=-+
  Add2 : Sum  Inputs=+-
  Add5 : Sum  Inputs=+++
  Add7 : Sum  Inputs=+-
  Add9 : Sum  Inputs=+++
  Constant : Constant  Value=0.75
  Constant1 : Constant  Value=0.85
  Constant2 : Constant  Value=0.8
  Constant3 : Constant  Value=0.8
  Constant4 : Constant  Value=0.5
  Constant5 : Constant  Value=1.5
  Constant6 : Constant  Value=0.5
  Constant7 : Constant  Value=1.5
  Gain : Gain  Gain=-1
  Product{1,3..9} (8 alike) : Product
  p3z : Outport
  wires:
  Product8/1 -> Add9/2
  Product9/1 -> Add9/3
  Constant2/1 -> Product8/1
  Add8/1 -> Product8/2
  vz3/1 -> Add6/2, Add8/2, Add7/1
  Constant6/1 -> Product9/2
  Add7/1 -> Product9/1
  vz4/1 -> Add8/1
  vz1/1 -> Add7/2
  vz5/1 -> Add6/1
  Constant7/1 -> Product7/1
  Add6/1 -> Product7/2
  Product7/1 -> Add9/1
  Product3/1 -> Add5/1
  Add1/1 -> Product3/2
  Constant5/1 -> Product3/1
  xz5/1 -> Add1/1
  xz1/1 -> Add2/2
  xz4/1 -> Add4/1
  Add5/1 -> Product6/2
  Add2/1 -> Product5/1
  Product1/1 -> Add/2
  Constant1/1 -> Product1/1
  Constant/1 -> Product6/1
  Product6/1 -> Add/1
  Constant4/1 -> Product5/2
  xz3/1 -> Add2/1, Add4/2, Add1/2
  Add4/1 -> Product4/2
  Constant3/1 -> Product4/1
  Product5/1 -> Add5/3
  Product4/1 -> Add5/2
  Add9/1 -> Product1/2
  Gain/1 -> p3z/1
  Add/1 -> Gain/1

== system chap05/Subsystem16/Subsystem5/Subsystem3 ==
  utx : Inport
  vx : Inport  Port=2
  vy : Inport  Port=3
  vz : Inport  Port=4
  uty : Inport  Port=5
  ux : Inport  Port=6
  uy : Inport  Port=7
  uz : Inport  Port=8
  utz : Inport  Port=9
  switch : Inport  Port=10
  Add3 : Sum  Inputs=-+
  Add4 : Sum  Inputs=-+
  Add5 : Sum  Inputs=-+
  Demux : Demux  Outputs=3
  Demux1 : Demux  Outputs=3
  Discrete-Time Integrator1 : DiscreteIntegrator  SampleTime=-1  ICPrevOutput=DiscIntNeverNeededParam  ICPrevScaledInput=DiscIntNeverNeededParam
  Discrete-Time Integrator2 : DiscreteIntegrator  SampleTime=-1  ICPrevOutput=DiscIntNeverNeededParam  ICPrevScaledInput=DiscIntNeverNeededParam
  Discrete-Time Integrator8 : DiscreteIntegrator  SampleTime=-1  ICPrevOutput=DiscIntNeverNeededParam  ICPrevScaledInput=DiscIntNeverNeededParam
  MATLAB Function : MATLAB Function  TreatAsAtomicUnit=on
  MATLAB Function1 : MATLAB Function  TreatAsAtomicUnit=on
  MATLAB Function2 : MATLAB Function  TreatAsAtomicUnit=on
  Mux : Mux  Inputs=3
  Mux1 : Mux  Inputs=3
  Subsystem : Subsystem
  Subsystem1 : Subsystem
  Subsystem2 : Subsystem
      settings: PortSchema="{\"entries\":[{\"content\":{\"sides\":[{\"content\":{\"connectorIds\":[\"In1\"]},\"type\":\"ConnectorPlacement.EquallySpacedRectSide\",\"uuid\":\"fc08b57d-5108-4bb3-894e-d1527c9ee9b9\"},{\"content\":{\"connectorIds\":[\"Out1\",\"Out2\",\"Out3\",\"Out4\"],\"side\":\"RIGHT\"},\"type\":\"ConnectorPlacement.EquallySpacedRectSide\",\"uuid\":\"5f28f464-9d6d-4ee7-848e-113b4b51ead6\"},{\"content\":{\"connectorIds\":[],\"side\":\"TOP\"},\"type\":\"ConnectorPlacement.EquallySpacedRectSide\",\"uuid\":\"5cca314e-822b-43eb-ac4d-78622e8ed582\"},{\"content\":{\"connectorIds\":[\"In2\"],\"side\":\"BOTTOM\"},\"type\":\"ConnectorPlacement.EquallySpacedRectSide\",\"uuid\":\"aa07b2d0-4f6e-4d8e-96de-14c35ee3da88\"}]},\"type\":\"ConnectorPlacement.EquallySpacedConnector\",\"uuid\":\"246d6f2c-2f9e-403c-b810-eff9b0fc0735\"}],\"packageUris\":[\"http://schema.mathworks.com/mf0/Connector/R2020b\"],\"version\":\"1.0\"}"
  Subsystem3 : Subsystem
  Subtract1 : Sum  Inputs=++++
  Subtract2 : Sum  Inputs=+-
  Subtract3 : Sum  Inputs=+-
  Subtract4 : Sum  Inputs=+-
  Switch1 : Switch  Criteria=u2 > Threshold  Threshold=1
  Switch2 : Switch  Criteria=u2 > Threshold  Threshold=1
  Switch3 : Switch  Criteria=u2 > Threshold  Threshold=1
  udtx : Outport
  udty : Outport  Port=2
  udtz : Outport  Port=3
  wires:
  Subsystem3/1(Out1) -> Subtract1/2
  Subsystem2/2(k2) -> Subsystem3/2(k2)
  Subsystem1/1(Out1) -> Subtract1/1
  Subsystem2/1(k1) -> Subsystem1/2(k1)
  Subtract4/1 -> MATLAB Function2/1(u)
  Subtract3/1 -> MATLAB Function1/1(u)
  Subtract2/1 -> MATLAB Function/1(u)
  Demux/3 -> Discrete-Time Integrator8/1
  Demux/1 -> Discrete-Time Integrator2/1
  Demux/2 -> Discrete-Time Integrator1/1
  Discrete-Time Integrator2/1 -> Subtract2/1
  Discrete-Time Integrator1/1 -> Subtract3/1
  Discrete-Time Integrator8/1 -> Subtract4/1
  Mux1/1 -> Subtract1/4
  ux/1 -> Mux1/1
  uy/1 -> Mux1/2
  uz/1 -> Mux1/3
  vx/1 -> Subtract2/2
  Subsystem2/4(k4) -> Subsystem/3(k4)
  Subsystem/1(z2) -> Subtract1/3, Demux1/1  "od3"
  Subsystem2/3(k3) -> Subsystem/2(k3)
  Subtract1/1 -> Demux/1
  Mux/1 -> Subsystem1/1(e1), Subsystem3/1(e1), Subsystem2/1(e1), Subsystem/1(e1)
  utx/1 -> Switch1/3, Add3/2
  uty/1 -> Switch2/3, Add5/2
  utz/1 -> Switch3/3, Add4/2
  vy/1 -> Subtract3/2
  vz/1 -> Subtract4/2
  MATLAB Function/1(y) -> Mux/1
  MATLAB Function1/1(y) -> Mux/2
  MATLAB Function2/1(y) -> Mux/3
  switch/1 -> [switch], Switch3/2, Switch2/2, Switch1/2
  [switch] -> Subsystem2/2(switch)
  Add3/1 -> Switch1/1
  Add5/1 -> Switch2/1
  Add4/1 -> Switch3/1
  Switch1/1 -> udtx/1
  Switch2/1 -> udty/1
  Switch3/1 -> udtz/1
  Demux1/1 -> Add3/1
  Demux1/2 -> Add5/1
  Demux1/3 -> Add4/1

== system chap05/Subsystem16/Subsystem5/Subsystem4 ==
  vx3 : Inport
  utx : Inport  Port=2
  gain : Inport  Port=3
  switch : Inport  Port=4
  Add1 : Sum  Inputs=--+
  Constant1 : Constant  Value=0.08
  Constant2 : Constant  Value=10
  Product : Product
  Product1 : Product
  Product2 : Product
  Subsystem : Subsystem
  Subtract : Sum  Inputs=+-
  Switch1 : Switch  Criteria=u2 > Threshold  Threshold=1
  Tanh : Trigonometry  Operator=tanh
  ux : Outport
  Sx : Outport  Port=2
  wires:
  Add1/1 -> Switch1/1
  utx/1 -> [A], Subsystem/2(zt3)
  Product/1 -> Add1/2
  vx3/1 -> Subtract/1
  Product2/1 -> Tanh/1
  Tanh/1 -> Product/1
  gain/1 -> Product/2
  [A] -> Add1/3
  Constant2/1 -> Product2/2
  Product1/1 -> Add1/1
  Constant1/1 -> Product1/1
  Subtract/1 -> Sx/1, Product1/2, Product2/1
  switch/1 -> [switch], Subsystem/1(switch)
  [A] -> Switch1/3
  [switch] -> Switch1/2
  Switch1/1 -> ux/1
  Subsystem/1(Out1) -> Subtract/2

== system chap05/Subsystem16/Subsystem5/Subsystem6 ==
  xx3 : Inport
  xx1 : Inport  Port=2
  xx4 : Inport  Port=3
  xx5 : Inport  Port=4
  vx3 : Inport  Port=5
  vx1 : Inport  Port=6
  vx4 : Inport  Port=7
  vx5 : Inport  Port=8
  Add : Sum
  Add{1,4,6,8} (4 alike) : Sum  Inputs=-+
  Add2 : Sum  Inputs=+-
  Add5 : Sum  Inputs=+++
  Add7 : Sum  Inputs=+-
  Add9 : Sum  Inputs=+++
  Constant : Constant  Value=0.75
  Constant1 : Constant  Value=0.85
  Constant2 : Constant  Value=0.8
  Constant3 : Constant  Value=0.8
  Constant4 : Constant  Value=0.5
  Constant5 : Constant  Value=1.5
  Constant6 : Constant  Value=0.5
  Constant7 : Constant  Value=1.5
  Gain : Gain  Gain=-1
  Product{1,3..9} (8 alike) : Product
  p3x : Outport
  wires:
  Product8/1 -> Add9/2
  Product9/1 -> Add9/3
  Constant2/1 -> Product8/1
  Add8/1 -> Product8/2
  vx3/1 -> Add6/2, Add8/2, Add7/1
  Constant6/1 -> Product9/2
  Add7/1 -> Product9/1
  vx4/1 -> Add8/1
  vx1/1 -> Add7/2
  vx5/1 -> Add6/1
  Constant7/1 -> Product7/1
  Add6/1 -> Product7/2
  Product7/1 -> Add9/1
  Product3/1 -> Add5/1
  Add1/1 -> Product3/2
  Constant5/1 -> Product3/1
  xx5/1 -> Add1/1
  xx1/1 -> Add2/2
  xx4/1 -> Add4/1
  Add5/1 -> Product6/2
  Add2/1 -> Product5/1
  Product1/1 -> Add/2
  Constant1/1 -> Product1/1
  Constant/1 -> Product6/1
  Product6/1 -> Add/1
  Constant4/1 -> Product5/2
  xx3/1 -> Add2/1, Add4/2, Add1/2
  Add4/1 -> Product4/2
  Constant3/1 -> Product4/1
  Product5/1 -> Add5/3
  Product4/1 -> Add5/2
  Add9/1 -> Product1/2
  Gain/1 -> p3x/1
  Add/1 -> Gain/1

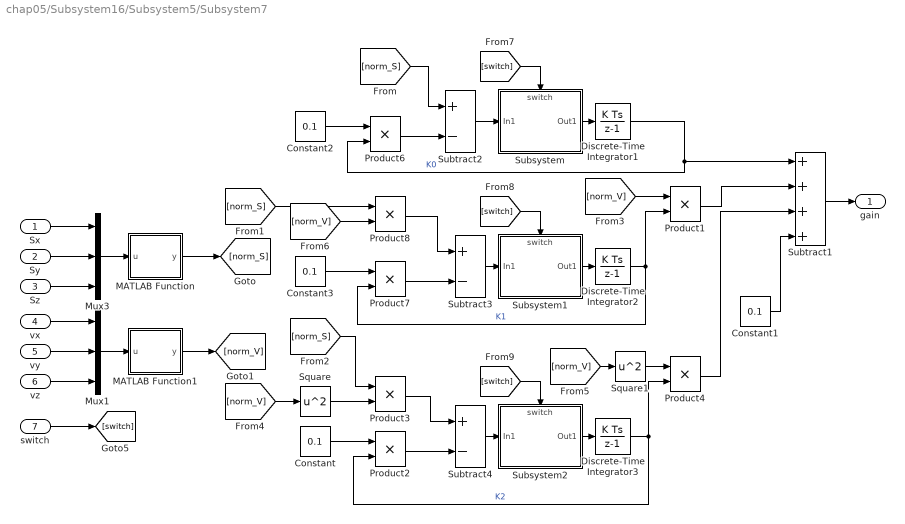
== system chap05/Subsystem16/Subsystem5/Subsystem7 ==
  Sx : Inport
  Sy : Inport  Port=2
  Sz : Inport  Port=3
  vx : Inport  Port=4
  vy : Inport  Port=5
  vz : Inport  Port=6
  switch : Inport  Port=7
  Constant{,1..3} (4 alike) : Constant  Value=0.1
  Discrete-Time Integrator1 : DiscreteIntegrator  gainval=1  InitialCondition=0.05  SampleTime=-1  ICPrevOutput=DiscIntNeverNeededParam  ICPrevScaledInput=DiscIntNeverNeededParam
  Discrete-Time Integrator2 : DiscreteIntegrator  gainval=1  InitialCondition=0.025  SampleTime=-1  ICPrevOutput=DiscIntNeverNeededParam  ICPrevScaledInput=DiscIntNeverNeededParam
  Discrete-Time Integrator3 : DiscreteIntegrator  gainval=1  InitialCondition=0.01  SampleTime=-1  ICPrevOutput=DiscIntNeverNeededParam  ICPrevScaledInput=DiscIntNeverNeededParam
  MATLAB Function : MATLAB Function  TreatAsAtomicUnit=on
  MATLAB Function1 : MATLAB Function  TreatAsAtomicUnit=on
  Mux1 : Mux  Inputs=3
  Mux3 : Mux  Inputs=3
  Product{1..4,6..8} (7 alike) : Product
  Square : Math  Operator=square  SaturateOnIntegerOverflow=on
  Square1 : Math  Operator=square  SaturateOnIntegerOverflow=on
  Subsystem : Subsystem
      settings: PortSchema="{\"entries\":[{\"content\":{\"sides\":[{\"content\":{\"connectorIds\":[\"In1\"]},\"type\":\"ConnectorPlacement.EquallySpacedRectSide\",\"uuid\":\"50b1559e-7173-4ba8-93e6-314f6d9df527\"},{\"content\":{\"connectorIds\":[\"Out1\"],\"side\":\"RIGHT\"},\"type\":\"ConnectorPlacement.EquallySpacedRectSide\",\"uuid\":\"be527bac-0bcc-4faf-a185-0382edae0189\"},{\"content\":{\"connectorIds\":[\"In2\"],\"side\":\"TOP\"},\"type\":\"ConnectorPlacement.EquallySpacedRectSide\",\"uuid\":\"4c8ef68d-7cf5-4d15-9758-89dbc1169805\"}]},\"type\":\"ConnectorPlacement.EquallySpacedConnector\",\"uuid\":\"3c2ee67b-c3c9-431a-8107-6d5cd22b236e\"}],\"packageUris\":[\"http://schema.mathworks.com/mf0/Connector/R2020b\"],\"version\":\"1.0\"}"
  Subsystem1 : Subsystem
      settings: PortSchema="{\"entries\":[{\"content\":{\"sides\":[{\"content\":{\"connectorIds\":[\"In1\"]},\"type\":\"ConnectorPlacement.EquallySpacedRectSide\",\"uuid\":\"50b1559e-7173-4ba8-93e6-314f6d9df527\"},{\"content\":{\"connectorIds\":[\"Out1\"],\"side\":\"RIGHT\"},\"type\":\"ConnectorPlacement.EquallySpacedRectSide\",\"uuid\":\"be527bac-0bcc-4faf-a185-0382edae0189\"},{\"content\":{\"connectorIds\":[\"In2\"],\"side\":\"TOP\"},\"type\":\"ConnectorPlacement.EquallySpacedRectSide\",\"uuid\":\"4c8ef68d-7cf5-4d15-9758-89dbc1169805\"}]},\"type\":\"ConnectorPlacement.EquallySpacedConnector\",\"uuid\":\"3c2ee67b-c3c9-431a-8107-6d5cd22b236e\"}],\"packageUris\":[\"http://schema.mathworks.com/mf0/Connector/R2020b\"],\"version\":\"1.0\"}"
  Subsystem2 : Subsystem
      settings: PortSchema="{\"entries\":[{\"content\":{\"sides\":[{\"content\":{\"connectorIds\":[\"In1\"]},\"type\":\"ConnectorPlacement.EquallySpacedRectSide\",\"uuid\":\"50b1559e-7173-4ba8-93e6-314f6d9df527\"},{\"content\":{\"connectorIds\":[\"Out1\"],\"side\":\"RIGHT\"},\"type\":\"ConnectorPlacement.EquallySpacedRectSide\",\"uuid\":\"be527bac-0bcc-4faf-a185-0382edae0189\"},{\"content\":{\"connectorIds\":[\"In2\"],\"side\":\"TOP\"},\"type\":\"ConnectorPlacement.EquallySpacedRectSide\",\"uuid\":\"4c8ef68d-7cf5-4d15-9758-89dbc1169805\"}]},\"type\":\"ConnectorPlacement.EquallySpacedConnector\",\"uuid\":\"3c2ee67b-c3c9-431a-8107-6d5cd22b236e\"}],\"packageUris\":[\"http://schema.mathworks.com/mf0/Connector/R2020b\"],\"version\":\"1.0\"}"
  Subtract1 : Sum  Inputs=++++
  Subtract2 : Sum  Inputs=+-
  Subtract3 : Sum  Inputs=+-
  Subtract4 : Sum  Inputs=+-
  " gain" : Outport
  wires:
  [switch] -> Subsystem2/2(switch)
  [switch] -> Subsystem1/2(switch)
  [switch] -> Subsystem/2(switch)
  switch/1 -> [switch]
  Subsystem1/1(Out1) -> Discrete-Time Integrator2/1
  Subsystem2/1(Out1) -> Discrete-Time Integrator3/1
  Subsystem/1(Out1) -> Discrete-Time Integrator1/1
  [norm_V] -> Product8/2
  Square1/1 -> Product4/1
  [norm_V] -> Square1/1
  [norm_V] -> Product1/1
  [norm_V] -> Square/1
  [norm_S] -> Product3/1
  [norm_S] -> Product8/1
  [norm_S] -> Subtract2/1
  MATLAB Function/1(y) -> [norm_S]
  vy/1 -> Mux1/2
  vz/1 -> Mux1/3
  vx/1 -> Mux1/1
  Sz/1 -> Mux3/3
  Sy/1 -> Mux3/2
  Sx/1 -> Mux3/1
  Constant3/1 -> Product7/1
  Constant2/1 -> Product6/1
  Constant1/1 -> Subtract1/4
  Product4/1 -> Subtract1/3
  MATLAB Function1/1(y) -> [norm_V]
  Constant/1 -> Product2/1
  Mux1/1 -> MATLAB Function1/1(u)
  Square/1 -> Product3/2
  Mux3/1 -> MATLAB Function/1(u)
  Discrete-Time Integrator3/1 -> Product2/2, Product4/2  "K2"
  Product2/1 -> Subtract4/2
  Product3/1 -> Subtract4/1
  Subtract4/1 -> Subsystem2/1(In1)
  Subtract1/1 -> " gain"/1
  Subtract3/1 -> Subsystem1/1(In1)
  Product8/1 -> Subtract3/1
  Product7/1 -> Subtract3/2
  Discrete-Time Integrator2/1 -> Product1/2, Product7/2  "K1"
  Product6/1 -> Subtract2/2
  Discrete-Time Integrator1/1 -> Subtract1/1, Product6/2  "K0"
  Subtract2/1 -> Subsystem/1(In1)
  Product1/1 -> Subtract1/2

== system chap05/Subsystem16/Subsystem5/Subsystem9 ==
  vy3 : Inport
  uty : Inport  Port=2
  gain : Inport  Port=3
  switch : Inport  Port=4
  Add1 : Sum  Inputs=--+
  Constant1 : Constant  Value=0.08
  Constant2 : Constant  Value=10
  Product : Product
  Product1 : Product
  Product2 : Product
  Subsystem : Subsystem
  Subtract : Sum  Inputs=+-
  Switch1 : Switch  Criteria=u2 > Threshold  Threshold=1
  Tanh : Trigonometry  Operator=tanh
  uy : Outport
  Sz : Outport  Port=2
  wires:
  Switch1/1 -> uy/1
  [switch] -> Switch1/2
  [A] -> Switch1/3
  switch/1 -> Subsystem/1(switch), [switch]
  Subtract/1 -> Product2/1, Product1/2, Sz/1
  Product1/1 -> Add1/1
  Constant2/1 -> Product2/2
  [A] -> Add1/3
  gain/1 -> Product/2
  Tanh/1 -> Product/1
  Product2/1 -> Tanh/1
  vy3/1 -> Subtract/1
  Product/1 -> Add1/2
  uty/1 -> Subsystem/2(zt3), [A]
  Add1/1 -> Switch1/1
  Subsystem/1(Out1) -> Subtract/2
  Constant1/1 -> Product1/1

== system chap05/Subsystem16/Subsystem6/Subsystem1 ==
  xx6 : Inport
  xx0 : Inport  Port=2
  xx1 : Inport  Port=3
  xx2 : Inport  Port=4
  vx6 : Inport  Port=5
  vx0 : Inport  Port=6
  vx1 : Inport  Port=7
  vx2 : Inport  Port=8
  Add : Sum
  Add1 : Sum  Inputs=-+
  Add10 : Sum  Inputs=-+
  Add2 : Sum  Inputs=+-
  Add4 : Sum  Inputs=-+
  Add5 : Sum  Inputs=+++
  Add6 : Sum  Inputs=+-
  Add8 : Sum  Inputs=+++
  Add9 : Sum  Inputs=+-
  Constant : Constant  Value=0.75
  Constant1 : Constant  Value=0.85
  Constant3 : Constant  Value=1.2
  Constant{4..5,7..8} (4 alike) : Constant  Value=1.5
  Constant6 : Constant  Value=1.2
  Gain : Gain  Gain=-1
  Product{1,3..9} (8 alike) : Product
  utx : Outport
  wires:
  Product7/1 -> Add8/3
  Add6/1 -> Product7/1
  Constant8/1 -> Product7/2
  vx0/1 -> Add6/2
  Product3/1 -> Add5/1
  Add1/1 -> Product3/2
  Constant7/1 -> Product3/1
  xx0/1 -> Add1/1
  vx6/1 -> Add10/2, Add9/1, Add6/1
  vx2/1 -> Add10/1
  vx1/1 -> Add9/2
  xx1/1 -> Add2/2
  xx2/1 -> Add4/1
  Add5/1 -> Product6/2
  Add2/1 -> Product5/1
  Product1/1 -> Add/2
  Constant1/1 -> Product1/1
  Constant/1 -> Product6/1
  Product6/1 -> Add/1
  Constant3/1 -> Product5/2
  xx6/1 -> Add4/2, Add2/1, Add1/2
  Add4/1 -> Product4/2
  Constant4/1 -> Product4/1
  Product5/1 -> Add5/3
  Product4/1 -> Add5/2
  Add8/1 -> Product1/2
  Constant5/1 -> Product8/1
  Add10/1 -> Product8/2
  Constant6/1 -> Product9/2
  Add9/1 -> Product9/1
  Product8/1 -> Add8/1
  Product9/1 -> Add8/2
  Gain/1 -> utx/1
  Add/1 -> Gain/1

== system chap05/Subsystem16/Subsystem6/Subsystem10 ==
  utx : Inport
  uty : Inport  Port=2
  utz : Inport  Port=3
  Add : Sum
  Constant3 : Constant
  Constant4 : Constant  Value=0
  Data Store Memory : DataStoreMemory  DataStoreName=utkz6  ReadBeforeWriteMsg=warning  WriteAfterWriteMsg=warning  WriteAfterReadMsg=warning  ShowAdditionalParam=off
  Data Store Memory1 : DataStoreMemory  DataStoreName=utky6  ReadBeforeWriteMsg=warning  WriteAfterWriteMsg=warning  WriteAfterReadMsg=warning  ShowAdditionalParam=off
  Data Store Memory2 : DataStoreMemory  DataStoreName=utkx6  ReadBeforeWriteMsg=warning  WriteAfterWriteMsg=warning  WriteAfterReadMsg=warning  ShowAdditionalParam=off
  Data Store Memory3 : DataStoreMemory  DataStoreName=uc6  ReadBeforeWriteMsg=warning  WriteAfterWriteMsg=warning  WriteAfterReadMsg=warning  ShowAdditionalParam=off
  Data Store Read : DataStoreRead  DataStoreName=uc6  IndexOptions=Index vector (dialog)  Indices=1  OutputSizes=1
  Data Store Read4 : DataStoreRead  DataStoreName=utkx6  IndexOptions=Index vector (dialog)  Indices=1  OutputSizes=1
  Data Store Read5 : DataStoreRead  DataStoreName=utky6  IndexOptions=Index vector (dialog)  Indices=1  OutputSizes=1
  Data Store Read6 : DataStoreRead  DataStoreName=utkz6  IndexOptions=Index vector (dialog)  Indices=1  OutputSizes=1
  Data Store Write : DataStoreWrite  DataStoreName=uc6  IndexOptions=Index vector (dialog)  Indices=1  OutputSizes=1
  Data Store Write1 : DataStoreWrite  DataStoreName=utkx6  IndexOptions=Index vector (dialog)  Indices=1  OutputSizes=1
  Data Store Write2 : DataStoreWrite  DataStoreName=utky6  IndexOptions=Index vector (dialog)  Indices=1  OutputSizes=1
  Data Store Write3 : DataStoreWrite  DataStoreName=utkz6  IndexOptions=Index vector (dialog)  Indices=1  OutputSizes=1
  Demux : Demux  Outputs=3
  Display : Display
  MATLAB Function : MATLAB Function  TreatAsAtomicUnit=on
  Mux1 : Mux  Inputs=3
  Mux2 : Mux  Inputs=3
  Switch : Switch  Threshold=0.1
  Switch2 : Switch  Threshold=0.1
  ux : Outport
  uy : Outport  Port=2
  uz : Outport  Port=3
  wires:
  Mux2/1 -> [utk], MATLAB Function/2(utk)
  Mux1/1 -> [ut], MATLAB Function/1(u)
  Switch/1 -> Demux/1
  Data Store Read4/1 -> Mux2/1
  Data Store Read6/1 -> Mux2/3
  Data Store Read5/1 -> Mux2/2
  Demux/3 -> Data Store Write3/1, uz/1
  Demux/1 -> Data Store Write1/1, ux/1
  Add/1 -> Display/1, Data Store Write/1
  Data Store Read/1 -> Add/2
  Switch2/1 -> Add/1  "e1"
  Constant3/1 -> Switch2/1
  Constant4/1 -> Switch2/3
  MATLAB Function/1(nrom) -> Switch2/2, Switch/2
  utx/1 -> Mux1/1
  uty/1 -> Mux1/2
  utz/1 -> Mux1/3
  Demux/2 -> Data Store Write2/1, uy/1
  [ut] -> Switch/1
  [utk] -> Switch/3

== system chap05/Subsystem16/Subsystem6/Subsystem2 ==
  xx6 : Inport
  xx0 : Inport  Port=2
  xx1 : Inport  Port=3
  xx2 : Inport  Port=4
  vx6 : Inport  Port=5
  vx0 : Inport  Port=6
  vx1 : Inport  Port=7
  vx2 : Inport  Port=8
  Add : Sum
  Add1 : Sum  Inputs=-+
  Add10 : Sum  Inputs=-+
  Add2 : Sum  Inputs=+-
  Add4 : Sum  Inputs=-+
  Add5 : Sum  Inputs=+++
  Add6 : Sum  Inputs=+-
  Add8 : Sum  Inputs=+++
  Add9 : Sum  Inputs=+-
  Constant : Constant  Value=0.75
  Constant1 : Constant  Value=0.85
  Constant3 : Constant  Value=1.2
  Constant{4..5,7..8} (4 alike) : Constant  Value=1.5
  Constant6 : Constant  Value=1.2
  Gain : Gain  Gain=-1
  Product{1,3..9} (8 alike) : Product
  utx : Outport
  wires:
  Product9/1 -> Add8/2
  Product8/1 -> Add8/1
  Add9/1 -> Product9/1
  Constant6/1 -> Product9/2
  Add10/1 -> Product8/2
  Constant5/1 -> Product8/1
  Add8/1 -> Product1/2
  Product4/1 -> Add5/2
  Product5/1 -> Add5/3
  Constant4/1 -> Product4/1
  Add4/1 -> Product4/2
  xx6/1 -> Add1/2, Add2/1, Add4/2
  Constant3/1 -> Product5/2
  Product6/1 -> Add/1
  Constant/1 -> Product6/1
  Constant1/1 -> Product1/1
  Product1/1 -> Add/2
  Add2/1 -> Product5/1
  Add5/1 -> Product6/2
  xx2/1 -> Add4/1
  xx1/1 -> Add2/2
  vx1/1 -> Add9/2
  vx2/1 -> Add10/1
  vx6/1 -> Add6/1, Add9/1, Add10/2
  xx0/1 -> Add1/1
  Constant7/1 -> Product3/1
  Add1/1 -> Product3/2
  Product3/1 -> Add5/1
  vx0/1 -> Add6/2
  Constant8/1 -> Product7/2
  Add6/1 -> Product7/1
  Product7/1 -> Add8/3
  Gain/1 -> utx/1
  Add/1 -> Gain/1
